simulink model "chap3_3sim"  (R2016b)
settings: Solver=ode45  StartTime=0.0  StopTime=10  FixedStep=0.01  RelTol=1e-3  EnableMultiTasking=on
settings Model: Creator=Masoud  LastModifiedBy=Hafez
settings DataIOCC: LimitDataPoints=on  SaveFormat=Array
settings OptimizationCC: LifeSpan=inf
settings DebuggingCC: InheritedTsInSrcMsg=none  SFUnexpectedBacktrackingDiag=warning  SFNoUnconditionalDefaultTransitionDiag=warning  SFExecutionAtInitializationDiag=none
settings HardwareCC: ProdBitPerPointer=32  ProdBitPerSizeT=32  ProdBitPerPtrDiffT=32  ProdLargestAtomicFloat=None  ProdIntDivRoundTo=Undefined  ProdEndianess=Unspecified  ProdWordSize=32  ProdHWDeviceType=32-bit Generic
settings ModelReferenceCC: PropagateSignalLabelsOutOfModel=off
settings GRTTargetCC: TargetLangStandard=C89/C90 (ANSI)  GeneratePreprocessorConditionals=Disable all
settings ConfigComp: CovMetricSettings=dw  CovHtmlReporting=on  CovSaveCumulativeToWorkspaceVar=on  CovSaveSingleToWorkspaceVar=on  CovExternalEMLEnable=off

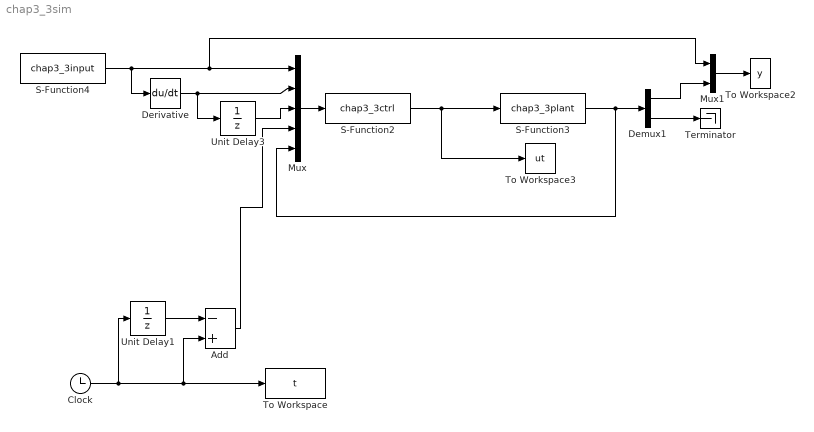
== system chap3_3sim ==
  Add : Sum  Inputs=-+
  Clock : Clock
  Demux1 : Demux  Outputs=2
  Derivative : Derivative
  Mux : Mux  Inputs=5
  Mux1 : Mux  Inputs=2
  S-Function2 : S-Function  FunctionName=chap3_3ctrl  SFunctionModules='chap3_3ctrl'  SFunctionDeploymentMode=off  EnableBusSupport=off
  S-Function3 : S-Function  FunctionName=chap3_3plant  SFunctionModules='chap3_3plant'  SFunctionDeploymentMode=off  EnableBusSupport=off
  S-Function4 : S-Function  FunctionName=chap3_3input  SFunctionModules='chap3_3nput'  SFunctionDeploymentMode=off  EnableBusSupport=off
  Terminator : Terminator
  To Workspace : ToWorkspace  VariableName=t  SampleTime=-1
  To Workspace2 : ToWorkspace  VariableName=y  SampleTime=-1
  To Workspace3 : ToWorkspace  VariableName=ut  SampleTime=-1
  Unit Delay1 : UnitDelay  SampleTime=-1
  Unit Delay3 : UnitDelay  SampleTime=-1
  wires:
  S-Function3/1 -> Mux/5, Demux1/1
  S-Function2/1 -> S-Function3/1, To Workspace3/1
  S-Function4/1 -> Derivative/1, Mux/1, Mux1/1
  Mux/1 -> S-Function2/1
  Demux1/1 -> Mux1/2
  Mux1/1 -> To Workspace2/1
  Demux1/2 -> Terminator/1
  Derivative/1 -> Unit Delay3/1, Mux/2
  Unit Delay3/1 -> Mux/3
  Clock/1 -> Unit Delay1/1, Add/2, To Workspace/1
  Unit Delay1/1 -> Add/1
  Add/1 -> Mux/4
